simulink model "replay"  (R2017a)
settings: Solver=FixedStepDiscrete  StartTime=0.0  StopTime=45  FixedStep=0.01  RelTol=1e-3
values from neighbouring files (symbols this model uses):
  data = cell2mat(data')    [plot_polysync_experiment.m]
undefined symbols (not defined in the file or in its folder): highway
settings Model: Creator=laptopuser  LastModifiedBy=laptopuser

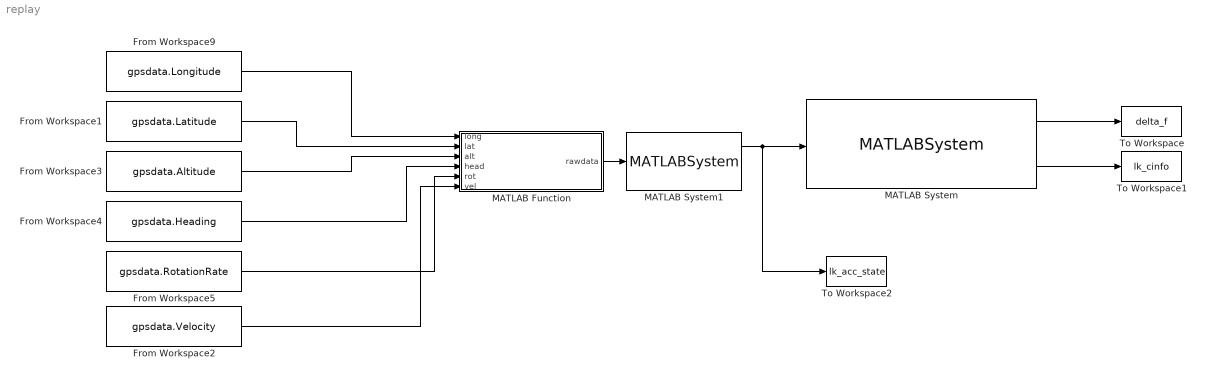
== system replay ==
  From Workspace1 : FromWorkspace  VariableName=gpsdata.Latitude  OutDataTypeStr=double  SampleTime=0
  From Workspace2 : FromWorkspace  VariableName=gpsdata.Velocity  OutDataTypeStr=double  SampleTime=0
  From Workspace3 : FromWorkspace  VariableName=gpsdata.Altitude  OutDataTypeStr=double  SampleTime=0
  From Workspace4 : FromWorkspace  VariableName=gpsdata.Heading  OutDataTypeStr=double  SampleTime=0
  From Workspace5 : FromWorkspace  VariableName=gpsdata.RotationRate  OutDataTypeStr=double  SampleTime=0
  From Workspace9 : FromWorkspace  VariableName=gpsdata.Longitude  OutDataTypeStr=double  SampleTime=0
  MATLAB Function : MATLAB Function  TreatAsAtomicUnit=on
  MATLAB System : MATLABSystem  System=lk_pcis_controller  M=1800  lf=1.2  lr=1.65  Caf=140000  Car=120000  Iz=3270  H_x=diag( [ 1, 0, 0.5, 0 ] )  f_x=zeros( 4, 1 )  H_u=2  f_u=0  sol_opts=struct( 'DataType', 'double', 'MaxIter', 200, 'FeasibilityTol', 1e-6, 'IntegrityChecks', true )  SimulateUsing=Code generation
      mask Type: lk_pcis_controller
      mask Display:
      | disp('lk_pcis_controller');
      | port_label('input',1,'lk_acc_state');
      | port_label('output',1,'delta_f');
      | port_label('output',2,'control_info');
  MATLAB System1 : MATLABSystem  System=road  lat0=42.30095833  long0=-83.69758056  h0=0  pathfile=data/run-highway.mat.ascii  circular=0  N_path=3  N_interp=10  dt=0.1  SimulateUsing=Code generation
      mask Type: road
      mask Display:
      | disp('road');
      | port_label('input',1,'data');
      | port_label('output',1,'lk_acc_state');
      | port_label('output',2,'road_left');
  To Workspace : ToWorkspace  VariableName=delta_f  SaveFormat=Timeseries  SampleTime=-1
  To Workspace1 : ToWorkspace  VariableName=lk_cinfo  SaveFormat=Timeseries  SampleTime=-1
  To Workspace2 : ToWorkspace  VariableName=lk_acc_state  SaveFormat=Timeseries  SampleTime=-1
  wires:
  MATLAB System/1 -> To Workspace/1
  MATLAB System/2 -> To Workspace1/1
  MATLAB System1/1 -> To Workspace2/1, MATLAB System/1
  MATLAB Function/1(rawdata) -> MATLAB System1/1
  From Workspace9/1 -> MATLAB Function/1(long)
  From Workspace1/1 -> MATLAB Function/2(lat)
  From Workspace3/1 -> MATLAB Function/3(alt)
  From Workspace4/1 -> MATLAB Function/4(head)
  From Workspace5/1 -> MATLAB Function/5(rot)
  From Workspace2/1 -> MATLAB Function/6(vel)

== matlab function replay/MATLAB Function ==
  data: long input; rawdata output Bus: DataBus; lat input; alt input; head input; rot input; vel input
function rawdata = fcn(long, lat, alt, head, rot, vel)

    rawdata = struct();

    normDeg = @(x) pi-mod(pi-x, 2*pi);

    % vector GPS -> CG
    r_gps_cg = [.99; 0];                     

    % rotational speed
    omega = rot(3);

    % velocity at GPS
    v_gps = [vel(1);
             vel(2)];     
    
    % velocity at CG
    v_cg = v_gps + (r_gps_cg) * omega;

    rawdata.latitude = rad2deg(lat);	% latitude of GPS  (deg)
    rawdata.longitude = rad2deg(long);	% longitude of GPS (deg)
    rawdata.el = alt;					% altitude of GPS  (m)
    rawdata.Yaw = normDeg(head + pi/2);	% yaw angle        (rad)  -- 0 is east, positive counter-clockwise
    rawdata.YawRate = omega;                		% yaw rate         (rad/s)
    rawdata.Vx = v_cg(1);           				% velocity at CG, car x axis   (m/s)
    rawdata.Vy = v_cg(2);           				% velocity at CG, car y axis   (m/s)
    rawdata.x_gps_cg = r_gps_cg(1); 				% position of CG from GPS, car x axis (m)
    rawdata.y_gps_cg = r_gps_cg(2);					% position of CG from GPS, car y axis (m)
    rawdata.steer_L1 = 0;
    rawdata.steer_R1 = 0;
    rawdata.Alpha_L1 = 0;
    rawdata.Alpha_R1 = 0;
    rawdata.Fy_L1 = 0;
    rawdata.Fy_R1 = 0;
    rawdata.Fz_L1 = 0;
    rawdata.Fz_R1 = 0;
    rawdata.Fx  = 0;
    rawdata.Gear_CL = 0;
    rawdata.RGear_Tr = 0;
    rawdata.AV_Eng = 0;
    rawdata.Throttle = 0;
    rawdata.Throttle_Eng = 0;			
    rawdata.M_EngOut = 0;
    rawdata.AVy_L1 = 0;
    rawdata.AVy_L2 = 0;
    rawdata.AVy_R1 = 0;
    rawdata.AVy_R2 = 0;
    rawdata.My_Dr_L1 = 0;
    rawdata.My_Dr_L2 = 0;
    rawdata.My_Dr_R1 = 0;
    rawdata.My_Dr_R2 = 0;
    rawdata.F_pedal = 0;
    rawdata.Bk_pedal = 0;
